simulink model "model6_2"  (R2025a)
settings: Solver=VariableStepAuto  StartTime=0.0  StopTime=2000  RelTol=1e-3
values from neighbouring files (symbols this model uses):
  Tf = 1    [domaci6_1.m]
settings Model: Creator=neso  LastModifiedBy=Nenad

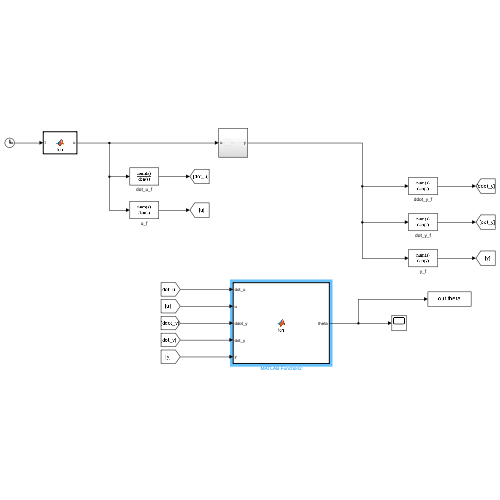
[thumbnail: Simulink's stored preview of the top-level diagram]
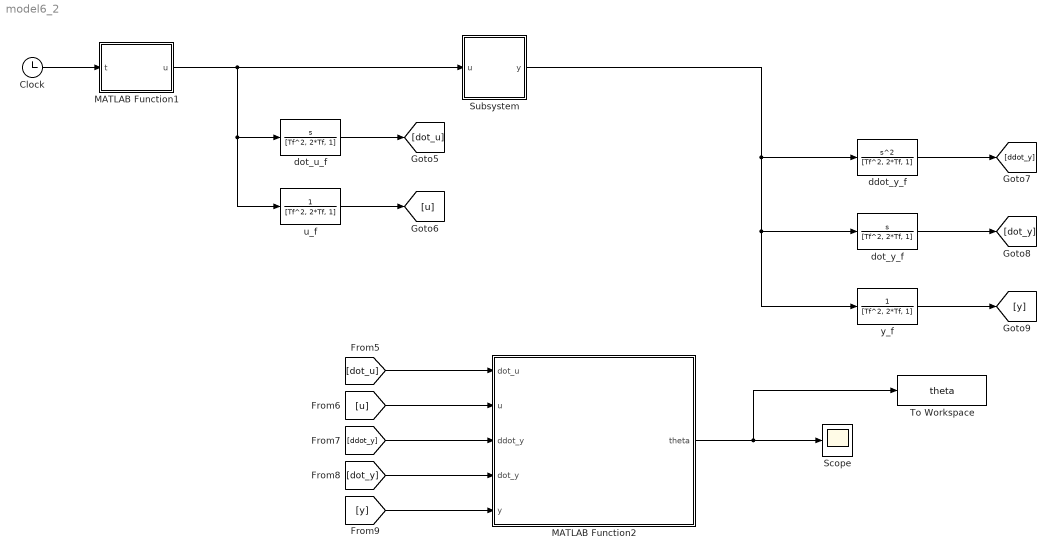
== system model6_2 ==
  Clock : Clock
  MATLAB Function1 : MATLAB Function  TreatAsAtomicUnit=on
  MATLAB Function2 : MATLAB Function  TreatAsAtomicUnit=on
  Scope : Scope
      settings: ActiveDisplayYMinimum=0.90722196048503356  ActiveDisplayYMaximum=4.7477253917762612
  Subsystem : Subsystem
  To Workspace : ToWorkspace  VariableName=theta  SaveFormat=Timeseries  SampleTime=-1
  ddot_y_f : TransferFcn  Numerator=[1, 0, 0]  Denominator=[Tf^2, 2*Tf, 1]
  dot_u_f : TransferFcn  Numerator=[1, 0]  Denominator=[Tf^2, 2*Tf, 1]
  dot_y_f : TransferFcn  Numerator=[1, 0]  Denominator=[Tf^2, 2*Tf, 1]
  u_f : TransferFcn  Numerator=1  Denominator=[Tf^2, 2*Tf, 1]
  y_f : TransferFcn  Numerator=1  Denominator=[Tf^2, 2*Tf, 1]
  wires:
  MATLAB Function1/1(u) -> u_f/1, dot_u_f/1, Subsystem/1(u)
  Subsystem/1(y) -> y_f/1, dot_y_f/1, ddot_y_f/1
  dot_u_f/1 -> [dot_u]
  u_f/1 -> [u]
  ddot_y_f/1 -> [ddot_y]
  dot_y_f/1 -> [dot_y]
  y_f/1 -> [y]
  [dot_u] -> MATLAB Function2/1(dot_u)
  [u] -> MATLAB Function2/2(u)
  [ddot_y] -> MATLAB Function2/3(ddot_y)
  [dot_y] -> MATLAB Function2/4(dot_y)
  [y] -> MATLAB Function2/5(y)
  MATLAB Function2/1(theta) -> Scope/1, To Workspace/1
  Clock/1 -> MATLAB Function1/1(t)

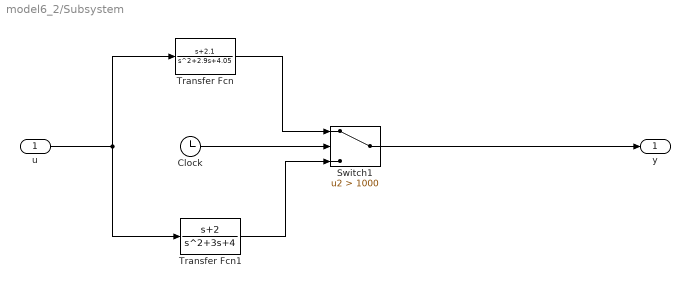
== system model6_2/Subsystem ==
  u : Inport
  Clock : Clock
  Switch1 : Switch  Criteria=u2 > Threshold  Threshold=1000  SaturateOnIntegerOverflow=off  InputSameDT=off
  Transfer Fcn : TransferFcn  Numerator=[1, 2.1]  Denominator=[1, 2.9, 4.05]
  Transfer Fcn1 : TransferFcn  Numerator=[1, 2]  Denominator=[1, 3, 4]
  y : Outport
  wires:
  Switch1/1 -> y/1
  u/1 -> Transfer Fcn1/1, Transfer Fcn/1
  Clock/1 -> Switch1/2
  Transfer Fcn/1 -> Switch1/1
  Transfer Fcn1/1 -> Switch1/3

== matlab function model6_2/MATLAB Function1 ==
  data: t input; u output
function u = fcn(t)
    u = 0;
    fmax = 10;
    for i = 1:fmax
        u = u + sin(2 * pi * i * t);
    end

== matlab function model6_2/MATLAB Function2 ==
  settings: updateMethod=DISCRETE  sampleTime=0.01
  data: dot_u input; u input; theta output; ddot_y input; dot_y input; y input
function theta = fcn(dot_u, u, ddot_y, dot_y, y)
    persistent P;
    persistent Theta;
    lambda = 0.999;
    
    phi = [-dot_y; -y; dot_u; u];
    eta = ddot_y;
    
    if isempty(Theta)
        Theta = zeros(length(phi), 1);
    end

    if isempty(P)
        P = 10000 * eye(length(phi), length(phi));
    end

    P = 1 / lambda * (P - (P * (phi * phi') * P) / (lambda + phi' * P * phi));
    
    Theta = Theta + P * phi * (eta - phi' * Theta);
    theta = Theta;
end
